simulink model "testFcn"  (R2022a)
settings: Solver=VariableStepAuto  StartTime=0.0  StopTime=365  RelTol=1e-3
libraries: simulink x1
settings Model: Creator=user  LastModifiedBy=user
settings SolverCC: AlgebraicLoopSolver=TrustRegion
settings DataIOCC: ReturnWorkspaceOutputs=off
settings DebuggingCC: UnconnectedInputMsg=warning  UnconnectedOutputMsg=warning  UnconnectedLineMsg=warning  SFMachineParentedDataDiag=warning  ArithmeticOperatorsInVariantConditions=warning
settings SFSimCC: CustomCodeUndefinedFunction=UseInterfaceOnly

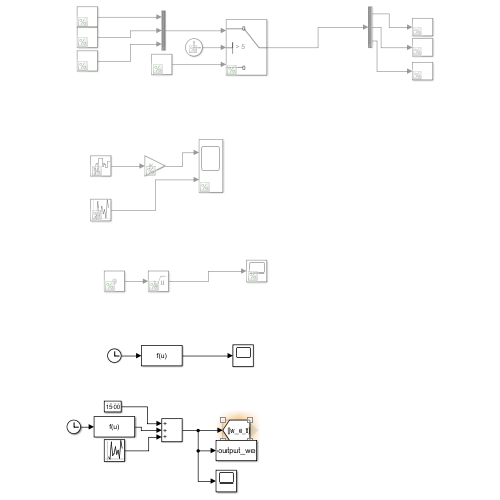
[thumbnail: Simulink's stored preview of the top-level diagram]
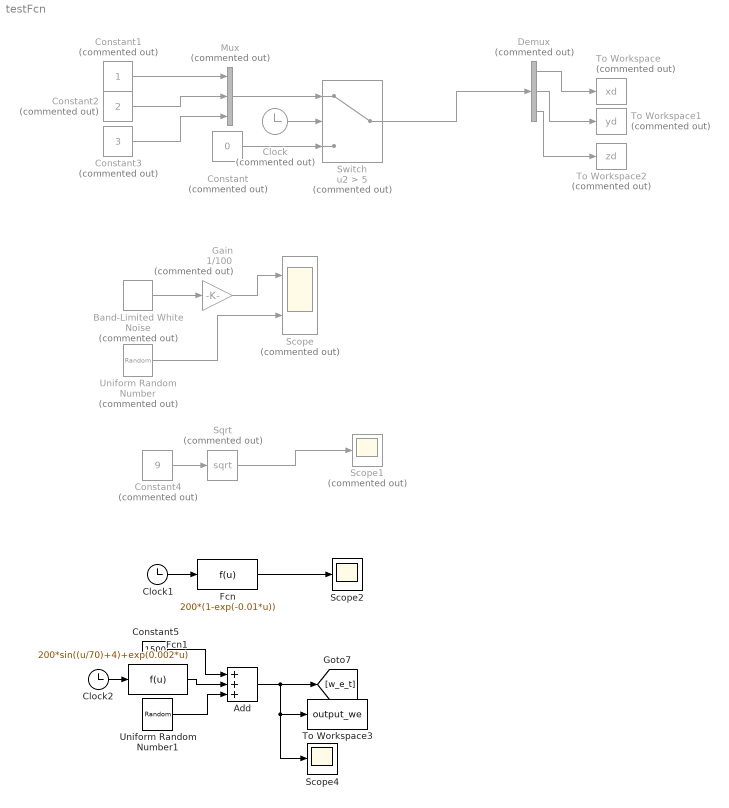
== system testFcn ==
  Add : Sum  Inputs=+++
  Band-Limited White Noise : simulink/Sources/Band-Limited White Noise  Commented=on  Cov=[0.1]  Ts=0.01  seed=[23341]
  Clock : Clock  Commented=on
      settings: Decimation=5
  Clock1 : Clock
  Clock2 : Clock
  Constant : Constant  Commented=on  Value=0
  Constant1 : Constant  Commented=on
  Constant2 : Constant  Commented=on  Value=2
  Constant3 : Constant  Commented=on  Value=3
  Constant4 : Constant  Commented=on  Value=9
  Constant5 : Constant  Value=1500
  Demux : Demux  Commented=on  Outputs=3
  Fcn : Fcn  Expr=200*(1-exp(-0.01*u))
  Fcn1 : Fcn  Expr=200*sin((u/70)+4)+exp(0.002*u)
  Gain : Gain  Commented=on  Gain=1/100
  Mux : Mux  Commented=on  Inputs=3
  Scope : Scope  Commented=on  NumInputPorts=2
  Scope1 : Scope  Commented=on
  Scope2 : Scope
  Scope4 : Scope
  Sqrt : Sqrt  Commented=on
  Switch : Switch  Commented=on  Criteria=u2 > Threshold  Threshold=5  SaturateOnIntegerOverflow=off  InputSameDT=off
  To Workspace : ToWorkspace  Commented=on  VariableName=xd  SampleTime=-1
  To Workspace1 : ToWorkspace  Commented=on  VariableName=yd  SampleTime=-1
  To Workspace2 : ToWorkspace  Commented=on  VariableName=zd  SampleTime=-1
  To Workspace3 : ToWorkspace  VariableName=output_we  SampleTime=0.1
  Uniform Random Number : UniformRandomNumber  Commented=on  Minimum=0  Maximum=0.1  SampleTime=0.01
  Uniform Random Number1 : UniformRandomNumber  Minimum=100  Maximum=500  SampleTime=80
  wires:
  Clock/1 -> Switch/2
  Switch/1 -> Demux/1
  Demux/1 -> To Workspace/1
  Demux/2 -> To Workspace1/1
  Demux/3 -> To Workspace2/1
  Constant1/1 -> Mux/1
  Constant2/1 -> Mux/2
  Constant3/1 -> Mux/3
  Mux/1 -> Switch/1
  Constant/1 -> Switch/3
  Gain/1 -> Scope/1
  Band-Limited White Noise/1 -> Gain/1
  Uniform Random Number/1 -> Scope/2
  Constant4/1 -> Sqrt/1
  Sqrt/1 -> Scope1/1
  Clock1/1 -> Fcn/1
  Fcn/1 -> Scope2/1
  Clock2/1 -> Fcn1/1
  Add/1 -> [w_e_t], Scope4/1, To Workspace3/1
  Fcn1/1 -> Add/2
  Constant5/1 -> Add/1
  Uniform Random Number1/1 -> Add/3
